simulink model "w1project8_2019a"  (R2019a)
settings: Solver=VariableStepAuto  StartTime=0.0  StopTime=10.0  RelTol=1e-3
settings Model: EnablePacing=on  PacingRate=0.200000  Creator=rutvi  LastModifiedBy=rutvi

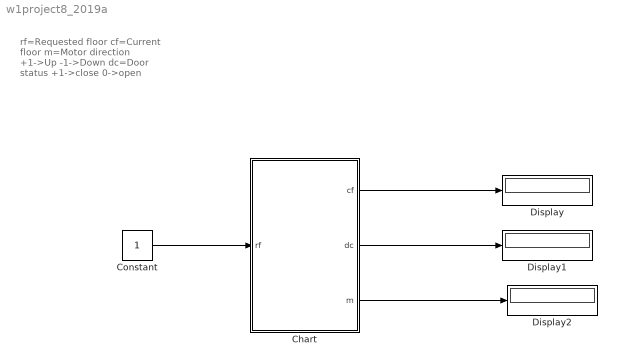
== system w1project8_2019a ==
  note: rf=Requested floor
      | cf=Current floor
      | m=Motor direction
      | +1->Up
      | -1->Down
      | dc=Door status
      | +1->close
      | 0->open
  Chart : Stateflow chart  TreatAsAtomicUnit=on
  Constant : Constant
  Display : Display
  Display1 : Display
  Display2 : Display
  wires:
  Constant/1 -> Chart/1(rf)
  Chart/1(cf) -> Display/1
  Chart/2(dc) -> Display1/1
  Chart/3(m) -> Display2/1

== stateflow chart w1project8_2019a/Chart ==
  state Elevator
    state Idle
      entry:m=0;
    state Door_closed
      entry:dc=1;
    state Down
      entry:m=-1;
      during:cf=cf-1;
    state Up
      entry:m=1;
      during:cf=cf+1;
    state Stop
      entry:m=0;dc=1;
      during:m=0;
    state Door_open
      entry:dc=0;
      during:dc=0;m=0;
    (default) -> Idle
    Idle -> Idle [order 2] : [rf==cf]
    Door_open -> Idle : after(2,sec)
    Idle -> Door_closed [order 1] : [rf~=cf]
    Door_closed -> Up [order 1] : [rf>cf]
    Door_closed -> Down [order 2] : [rf<cf]
    Down -> Stop : [rf==cf]
    Up -> Stop : [rf==cf]
    Stop -> Door_open : [rf==cf]
  (default) -> Elevator
  data: cf output =0; rf input; dc output =0; m output =0
